simulink model "PR_4_var15"  (R2020b)
settings: Solver=FixedStepAuto  StartTime=0.0  StopTime=10  FixedStep=0.01  RelTol=1e-3
libraries: simulink x2
settings Model: Creator=SIA  LastModifiedBy=SIA

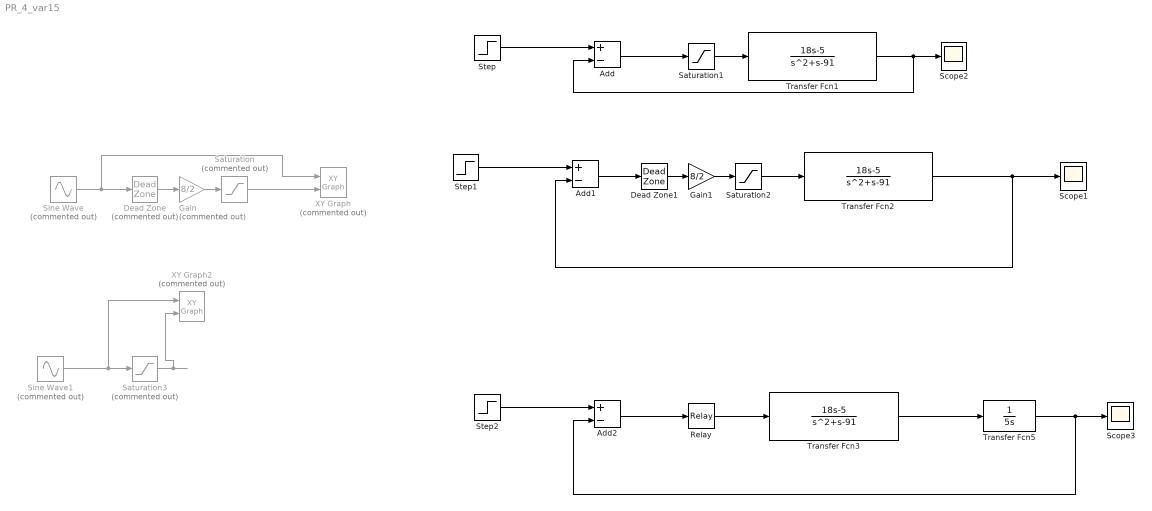
== system PR_4_var15 ==
  Add : Sum  Inputs=+-
  Add1 : Sum  Inputs=+-
  Add2 : Sum  Inputs=+-
  Dead Zone : DeadZone  Commented=on  LowerValue=-2  UpperValue=2  SaturateOnIntegerOverflow=on
  Dead Zone1 : DeadZone  LowerValue=-2  UpperValue=2  SaturateOnIntegerOverflow=on
  Gain : Gain  Commented=on  Gain=8/2
  Gain1 : Gain  Gain=8/2
  Relay : Relay  OnSwitchValue=3  OffSwitchValue=-3
  Saturation : Saturate  Commented=on  UpperLimit=8  LowerLimit=-8
  Saturation1 : Saturate  UpperLimit=5  LowerLimit=-5
  Saturation2 : Saturate  UpperLimit=8  LowerLimit=-8
  Saturation3 : Saturate  Commented=on  UpperLimit=5  LowerLimit=-5
  Scope1 : Scope
  Scope2 : Scope
  Scope3 : Scope
  Sine Wave : Sin  Commented=on  Amplitude=10  SampleTime=0
  Sine Wave1 : Sin  Commented=on  Amplitude=10  SampleTime=0
  Step : Step  Time=0  SampleTime=0
  Step1 : Step  Time=0  After=11  SampleTime=0
  Step2 : Step  Time=0  After=3  SampleTime=0
  Transfer Fcn1 : TransferFcn  Numerator=[18 -5]  Denominator=[1 1 -91]
  Transfer Fcn2 : TransferFcn  Numerator=[18 -5]  Denominator=[1 1 -91]
  Transfer Fcn3 : TransferFcn  Numerator=[18 -5]  Denominator=[1 1 -91]
  Transfer Fcn5 : TransferFcn  Denominator=[5 0]
  XY Graph : simulink/Sinks/XY Graph  Commented=on  xmin=-10  xmax=10  ymin=-10  ymax=10  st=-1
  XY Graph2 : simulink/Sinks/XY Graph  Commented=on  xmin=-10  xmax=10  ymin=-10  ymax=10  st=-1
  wires:
  Step/1 -> Add/1
  Add/1 -> Saturation1/1
  Saturation1/1 -> Transfer Fcn1/1
  Transfer Fcn1/1 -> Add/2, Scope2/1
  Step1/1 -> Add1/1
  Add1/1 -> Dead Zone1/1
  Transfer Fcn2/1 -> Scope1/1, Add1/2
  Saturation2/1 -> Transfer Fcn2/1
  Relay/1 -> Transfer Fcn3/1
  Transfer Fcn3/1 -> Transfer Fcn5/1
  Add2/1 -> Relay/1
  Transfer Fcn5/1 -> Scope3/1, Add2/2
  Step2/1 -> Add2/1
  Dead Zone/1 -> Gain/1
  Sine Wave/1 -> XY Graph/1, Dead Zone/1
  Saturation/1 -> XY Graph/2
  Gain/1 -> Saturation/1
  Dead Zone1/1 -> Gain1/1
  Gain1/1 -> Saturation2/1
  Sine Wave1/1 -> XY Graph2/1, Saturation3/1
  Saturation3/1 -> XY Graph2/2
